simulink model "SrmAmLinearApcZhw3a1tst UNKnwn"  (R2013b)
settings: Solver=ode45  StartTime=0.0  StopTime=2  MaxStep=1e-4  RelTol=1e-3
InitFcn:
  | theta0=30*2*pi/360;
  | ks=2.44;
  | is=2;
  | lu=0.016;
  | rs=5;
  | lux=1;
  | j=1;
settings Model: Creator=mamingkai  LastModifiedBy=Think79

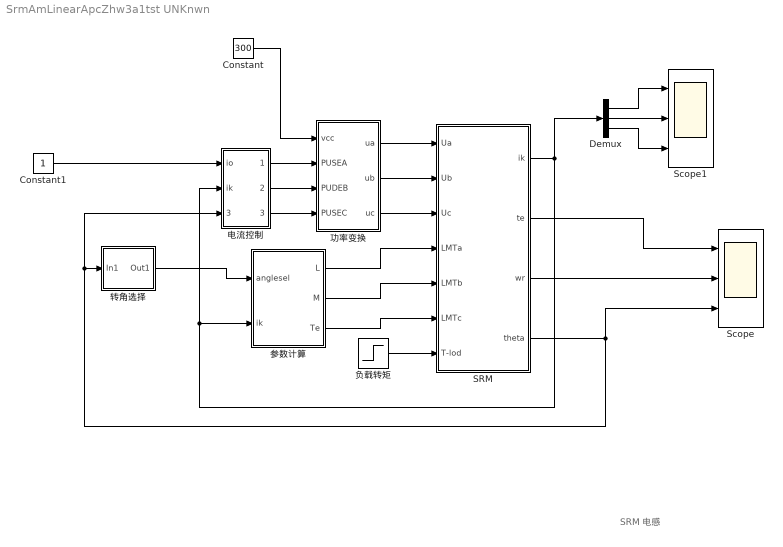
== system SrmAmLinearApcZhw3a1tst UNKnwn ==
  note: SRM 电感
  Constant : Constant  Value=300
  Constant1 : Constant
  Demux : Demux  Outputs=3
  SRM : Subsystem
  Scope : Scope  NumInputPorts=3
      settings: YMin=-5~-5~-5  YMax=5~5~5
  Scope1 : Scope  NumInputPorts=3
      settings: YMin=-5~-5~-5  YMax=5~5~5  SaveName=ScopeData6
  功率变换 : Subsystem
  参数计算 : Subsystem
  电流控制 : Subsystem
  负载转矩 : Step  After=0  SampleTime=0
  转角选择 : Subsystem
  wires:
  电流控制/1(Out1) -> 功率变换/2(PUSEA)
  电流控制/2(Out2) -> 功率变换/3(PUDEB)
  电流控制/3(Out3) -> 功率变换/4(PUSEC)
  Constant1/1 -> 电流控制/1(io)
  Constant/1 -> 功率变换/1(vcc)
  功率变换/1(ua) -> SRM/1(Ua)
  功率变换/2(ub) -> SRM/2(Ub)
  功率变换/3(uc) -> SRM/3(Uc)
  转角选择/1(Out1) -> 参数计算/1("anglesel ")
  SRM/1(ik) -> 电流控制/2(ik), 参数计算/2(ik), Demux/1
  SRM/3(wr) -> Scope/2
  SRM/4(theta) -> Scope/3, 电流控制/3(teta), 转角选择/1(In1)
  SRM/2(te) -> Scope/1
  参数计算/1(L) -> SRM/4(LMTa)
  参数计算/2(M) -> SRM/5(LMTb)
  参数计算/3(Te) -> SRM/6(LMTc)
  负载转矩/1 -> SRM/7(T-lod)
  Demux/1 -> Scope1/1
  Demux/2 -> Scope1/2
  Demux/3 -> Scope1/3

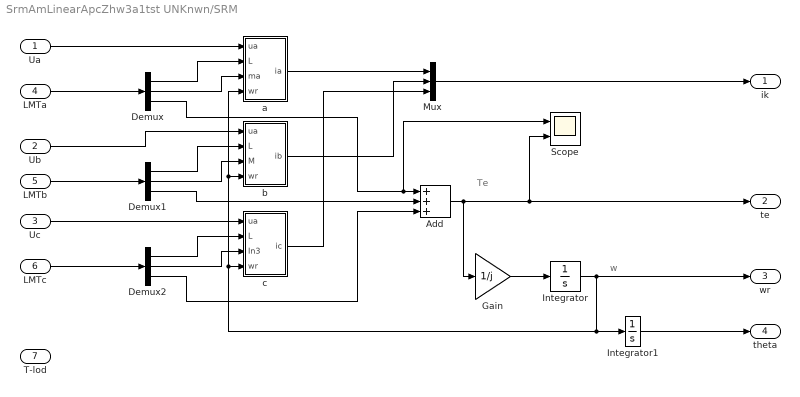
== system SrmAmLinearApcZhw3a1tst UNKnwn/SRM ==
  note: w
  note: Te
  Ua : Inport
  Ub : Inport  Port=2
  Uc : Inport  Port=3
  LMTa : Inport  Port=4
  LMTb : Inport  Port=5
  LMTc : Inport  Port=6
  T-lod : Inport  Port=7
  Add : Sum  Inputs=+++
  Demux : Demux  Outputs=3
  Demux1 : Demux  Outputs=3
  Demux2 : Demux  Outputs=3
  Gain : Gain  Gain=1/j
  Integrator : Integrator
  Integrator1 : Integrator
  Mux : Mux  Inputs=3
  Scope : Scope  NumInputPorts=2
      settings: YMin=-5~-5  YMax=5~5
  a : Subsystem
  b : Subsystem
  c : Subsystem
  ik : Outport
  te : Outport  Port=2
  wr : Outport  Port=3
  theta : Outport  Port=4
  wires:
  LMTa/1 -> Demux/1
  Demux/1 -> a/2("L ")
  Demux/2 -> a/3(ma)
  Demux/3 -> Scope/1, Add/1
  Ub/1 -> b/1(ua)
  Demux1/1 -> b/2(L)
  Demux1/2 -> b/3(M)
  Demux1/3 -> Add/2
  Uc/1 -> c/1(ua)
  LMTc/1 -> Demux2/1
  LMTb/1 -> Demux1/1
  Demux2/1 -> c/2(L)
  Demux2/2 -> c/3(In3)
  Demux2/3 -> Add/3
  Integrator/1 -> wr/1, c/4(wr), b/4("wr "), a/4(wr), Integrator1/1
  a/1(ia) -> Mux/1
  b/1("ib ") -> Mux/2
  c/1(ic) -> Mux/3
  Mux/1 -> ik/1
  Add/1 -> Gain/1, te/1, Scope/2
  Gain/1 -> Integrator/1
  Integrator1/1 -> theta/1
  Ua/1 -> a/1(ua)

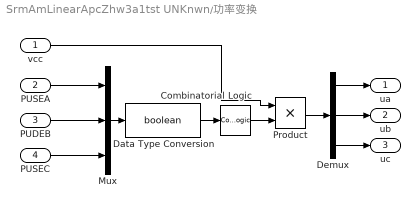
== system SrmAmLinearApcZhw3a1tst UNKnwn/功率变换 ==
  vcc : Inport
  PUSEA : Inport  Port=2
  PUDEB : Inport  Port=3
  PUSEC : Inport  Port=4
  Combinatorial Logic : CombinatorialLogic  TruthTable=[0 0 0 ;0 0 1;0 1 0;0 1 1;1 0 0;1 0 1;1 1 0;1 1 1]
  Data Type Conversion : DataTypeConversion  OutDataTypeStr=boolean
  Demux : Demux  Outputs=3
  Mux : Mux  Inputs=3
  Product : Product
  ua : Outport
  ub : Outport  Port=2
  uc : Outport  Port=3
  wires:
  PUSEA/1 -> Mux/1
  Demux/1 -> ua/1
  Product/1 -> Demux/1
  Demux/2 -> ub/1
  Demux/3 -> uc/1
  PUDEB/1 -> Mux/2
  PUSEC/1 -> Mux/3
  Combinatorial Logic/1 -> Product/2
  vcc/1 -> Product/1
  Mux/1 -> Data Type Conversion/1
  Data Type Conversion/1 -> Combinatorial Logic/1

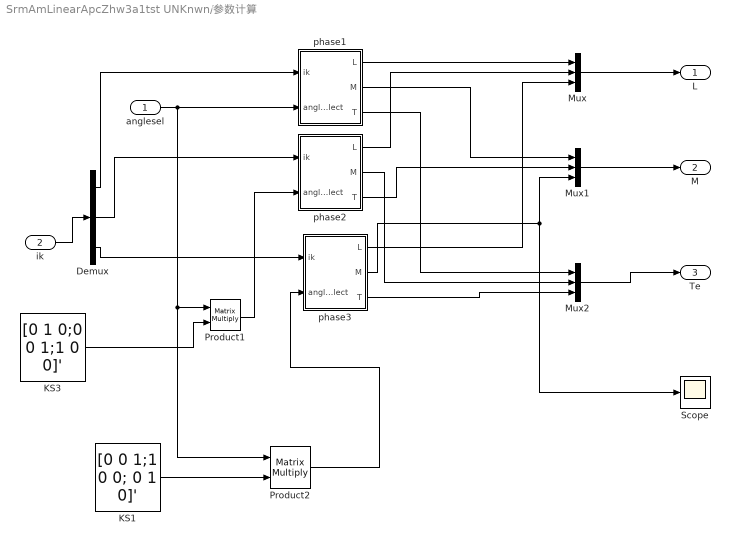
== system SrmAmLinearApcZhw3a1tst UNKnwn/参数计算 ==
  "anglesel " : Inport
  ik : Inport  Port=2
  Demux : Demux  Outputs=3
  KS1 : Constant  Value="[0 0 1;1 0  0; 0 1 0]'"  VectorParams1D=off
  KS3 : Constant  Value="[0 1 0;0  0 1;1 0 0]'"  VectorParams1D=off
  Mux : Mux  Inputs=3
  Mux1 : Mux  Inputs=3
  Mux2 : Mux  Inputs=3
  Product1 : Product  Multiplication=Matrix(*)
  Product2 : Product  Multiplication=Matrix(*)
  Scope : Scope
      settings: SaveName=ScopeData15
  phase1 : Subsystem
  phase2 : Subsystem
  phase3 : Subsystem
  L : Outport
  M : Outport  Port=2
  Te : Outport  Port=3
  wires:
  Mux/1 -> L/1
  "anglesel "/1 -> Product2/1, Product1/1, phase1/2("angleselect ")
  ik/1 -> Demux/1
  Demux/1 -> phase1/1(ik)
  Demux/2 -> phase2/1(ik)
  Demux/3 -> phase3/1(ik)
  phase1/1("L ") -> Mux/1
  phase1/2(M) -> Mux1/1
  phase1/3(T) -> Mux2/1
  phase2/1("L ") -> Mux/2
  phase2/3(T) -> Mux1/2
  phase2/2(M) -> Mux2/2
  phase3/1("L ") -> Mux/3
  phase3/2(M) -> Mux1/3, Scope/1
  phase3/3(T) -> Mux2/3
  Mux1/1 -> M/1
  Mux2/1 -> Te/1
  KS3/1 -> Product1/2
  Product1/1 -> phase2/2("angleselect ")
  KS1/1 -> Product2/2
  Product2/1 -> phase3/2("angleselect ")

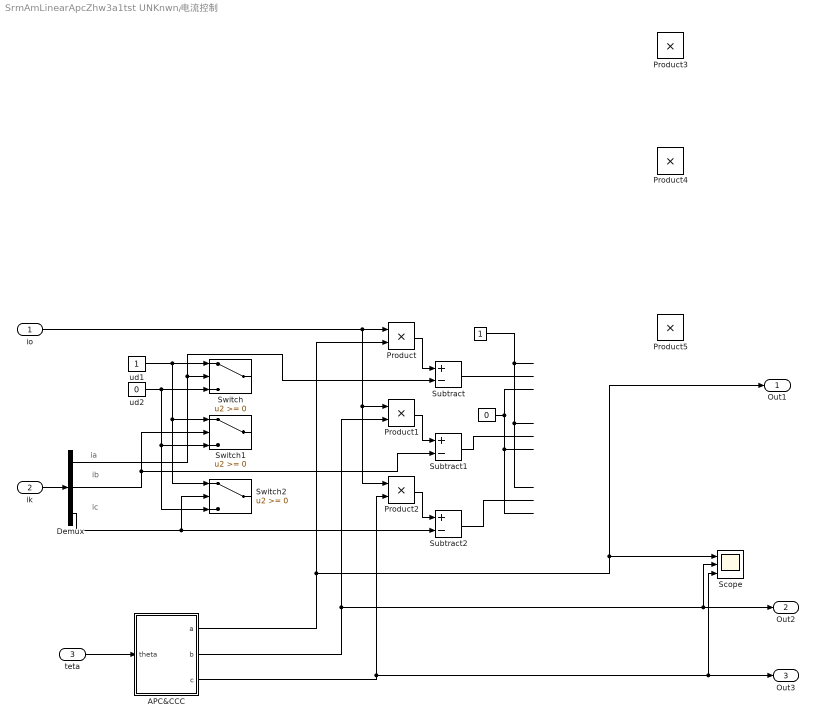
== system SrmAmLinearApcZhw3a1tst UNKnwn/电流控制 ==
  note: ic
  note: ib
  note: ia
  io : Inport
  ik : Inport  Port=2
  teta : Inport  Port=3
  " " : Constant
  " " : Constant  Value=0
  APC&CCC : Subsystem
  Demux : Demux  Outputs=3
  Product{,1..5} (6 alike) : Product
  Scope : Scope  NumInputPorts=3
      settings: YMin=-5~-5~-5  YMax=5~5~5  SaveName=ScopeData4
  Subtract : Sum  Inputs=+-
  Subtract1 : Sum  Inputs=+-
  Subtract2 : Sum  Inputs=+-
  Switch : Switch
  Switch1 : Switch
  Switch2 : Switch
  ud1 : Constant
  ud2 : Constant  Value=0
  Out1 : Outport
  Out2 : Outport  Port=2
  Out3 : Outport  Port=3
  wires:
  ik/1 -> Demux/1
  io/1 -> Product2/1, Product1/1, Product/1
  ud1/1 -> Switch2/1, Switch1/1, Switch/1
  ud2/1 -> Switch2/3, Switch1/3, Switch/3
  teta/1 -> APC&CCC/1(theta)
  Demux/1 -> Subtract/2, Switch/2
  Demux/3 -> Switch2/2, Subtract2/2
  Demux/2 -> Switch1/2, Subtract1/2
  APC&CCC/1(a) -> Out1/1, Scope/1, Product/2
  Product/1 -> Subtract/1
  Product1/1 -> Subtract1/1
  Product2/1 -> Subtract2/1
  " "/1 -> ?
  " "/1 -> ?
  ? -> Product5/1
  ? -> Product4/1
  ? -> Product3/1
  APC&CCC/3(c) -> Scope/3, Out3/1, Product2/2
  Subtract1/1 -> ?
  Subtract/1 -> ?
  Subtract2/1 -> ?
  APC&CCC/2(b) -> Scope/2, Out2/1, Product1/2

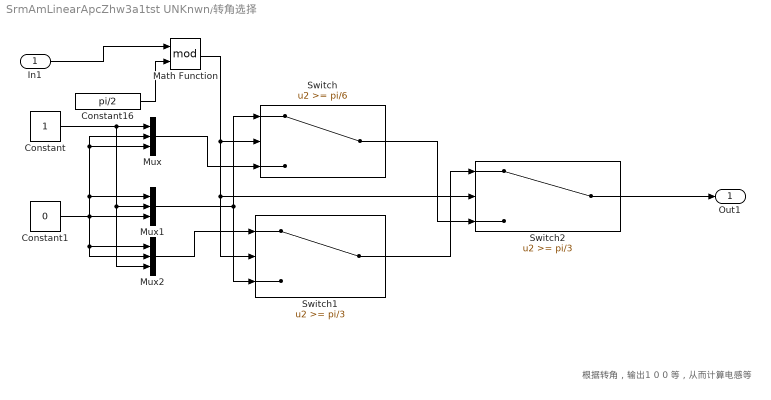
== system SrmAmLinearApcZhw3a1tst UNKnwn/转角选择 ==
  note: 根据转角，输出1 0 0 等，从而计算电感等
  In1 : Inport
  Constant : Constant
  Constant1 : Constant  Value=0
  Constant16 : Constant  Value=pi/2
  Math Function : Math  Operator=mod  SaturateOnIntegerOverflow=on
  Mux : Mux  Inputs=3
  Mux1 : Mux  Inputs=3
  Mux2 : Mux  Inputs=3
  Switch : Switch  Threshold=pi/6
  Switch1 : Switch  Threshold=pi/3
  Switch2 : Switch  Threshold=pi/3
  Out1 : Outport
  wires:
  In1/1 -> Math Function/1
  Constant/1 -> Mux2/3, Mux1/2, Mux/1
  Mux/1 -> Switch/3
  Constant1/1 -> Mux/3, Mux/2, Mux1/1, Mux2/2, Mux2/1, Mux1/3
  Mux1/1 -> Switch1/3, Switch/1
  Mux2/1 -> Switch1/1
  Math Function/1 -> Switch2/2, Switch1/2, Switch/2
  Switch/1 -> Switch2/3
  Switch1/1 -> Switch2/1
  Switch2/1 -> Out1/1
  Constant16/1 -> Math Function/2

== system SrmAmLinearApcZhw3a1tst UNKnwn/SRM/a ==
  ua : Inport
  "L " : Inport  Port=2
  ma : Inport  Port=3
  wr : Inport  Port=4
  Add : Sum  Inputs=+--
  Constant : Constant  Value=lux
  Gain : Gain  Gain=rs
  Integrator : Integrator
  Product : Product
  Product1 : Product
  Scope : Scope
      settings: SaveName=ScopeData2
  ia : Outport
  wires:
  wr/1 -> Product/2
  Integrator/1 -> Scope/1, Gain/1, ia/1
  ma/1 -> Product/1
  ua/1 -> Add/1
  Gain/1 -> Add/2
  Product/1 -> Add/3
  Add/1 -> Product1/1
  Product1/1 -> Integrator/1
  "L "/1 -> ?
  Constant/1 -> Product1/2

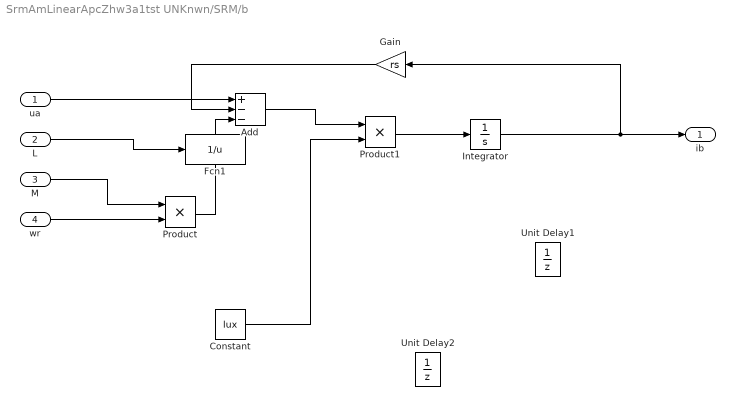
== system SrmAmLinearApcZhw3a1tst UNKnwn/SRM/b ==
  ua : Inport
  L : Inport  Port=2
  M : Inport  Port=3
  "wr " : Inport  Port=4
  Add : Sum  Inputs=+--
  Constant : Constant  Value=lux
  Fcn1 : Fcn  Expr=1/u
  Gain : Gain  Gain=rs
  Integrator : Integrator
  Product : Product
  Product1 : Product
  Unit Delay1 : UnitDelay  SampleTime=-1
  Unit Delay2 : UnitDelay  SampleTime=-1
  "ib " : Outport
  wires:
  "wr "/1 -> Product/2
  M/1 -> Product/1
  ua/1 -> Add/1
  Gain/1 -> Add/2
  Product/1 -> Add/3
  Add/1 -> Product1/1
  Product1/1 -> Integrator/1
  Integrator/1 -> Gain/1, "ib "/1
  L/1 -> Fcn1/1
  Constant/1 -> Product1/2

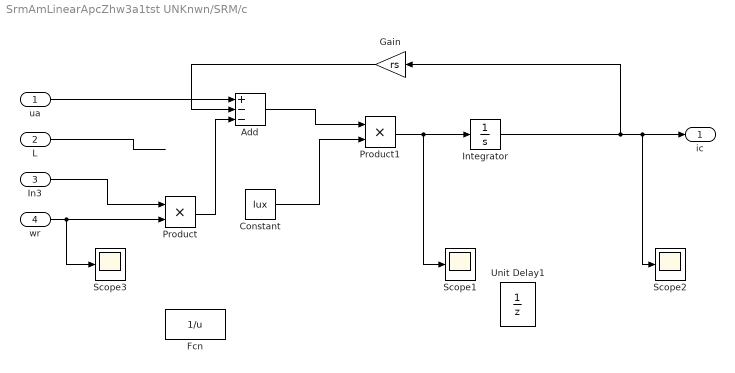
== system SrmAmLinearApcZhw3a1tst UNKnwn/SRM/c ==
  ua : Inport
  L : Inport  Port=2
  In3 : Inport  Port=3
  wr : Inport  Port=4
  Add : Sum  Inputs=+--
  Constant : Constant  Value=lux
  Fcn : Fcn  Expr=1/u
  Gain : Gain  Gain=rs
  Integrator : Integrator  InitialCondition=1e-5
  Product : Product
  Product1 : Product
  Scope1 : Scope
      settings: TimeRange=2  YMin=-1  YMax=1  SaveName=ScopeData13
  Scope2 : Scope
      settings: TimeRange=2  YMin=-1  YMax=1  SaveName=ScopeData12
  Scope3 : Scope
      settings: TimeRange=2  YMin=-1  YMax=1  SaveName=ScopeData14
  Unit Delay1 : UnitDelay  SampleTime=-1
  ic : Outport
  wires:
  wr/1 -> Scope3/1, Product/2
  In3/1 -> Product/1
  ua/1 -> Add/1
  Gain/1 -> Add/2
  Product/1 -> Add/3
  Add/1 -> Product1/1
  Integrator/1 -> Gain/1, Scope2/1, ic/1
  Product1/1 -> Scope1/1, Integrator/1
  L/1 -> ?
  Constant/1 -> Product1/2

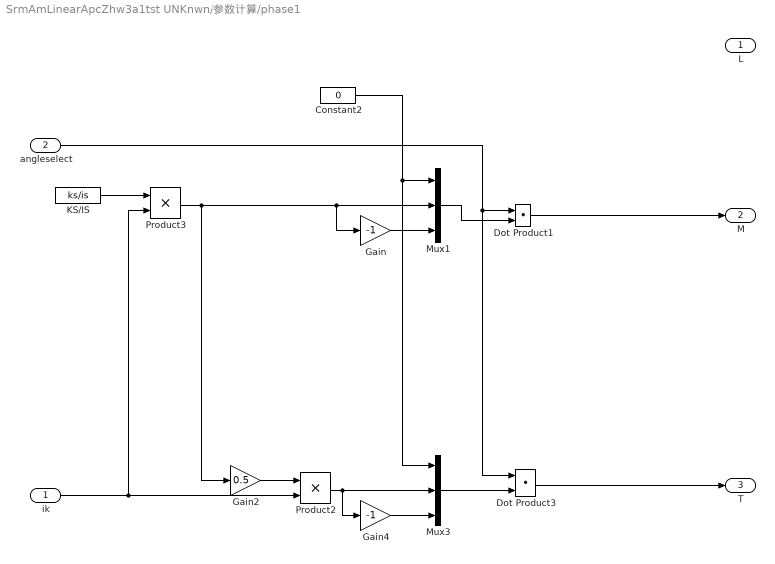
== system SrmAmLinearApcZhw3a1tst UNKnwn/参数计算/phase1 ==
  ik : Inport
  "angleselect " : Inport  Port=2
  Constant2 : Constant  Value=0
  Dot Product1 : DotProduct  InputSameDT=on  OutDataTypeStr=Inherit: Inherit via internal rule
  Dot Product3 : DotProduct  InputSameDT=on  OutDataTypeStr=Inherit: Inherit via internal rule
  Gain : Gain  Gain=-1
  Gain2 : Gain  Gain=0.5
  Gain4 : Gain  Gain=-1
  KS/IS : Constant  Value=ks/is
  Mux1 : Mux  Inputs=3
  Mux3 : Mux  Inputs=3
  Product2 : Product
  Product3 : Product
  "L " : Outport
  M : Outport  Port=2
  T : Outport  Port=3
  wires:
  ? -> "L "/1
  KS/IS/1 -> Product3/1
  ik/1 -> Product3/2, Product2/2
  "angleselect "/1 -> Dot Product3/1, Dot Product1/1
  Constant2/1 -> Mux3/1, Mux1/1
  Mux3/1 -> Dot Product3/2
  Mux1/1 -> Dot Product1/2
  Product3/1 -> Gain/1, Mux1/2, Gain2/1
  Gain/1 -> Mux1/3
  Gain2/1 -> Product2/1
  Dot Product1/1 -> M/1
  Dot Product3/1 -> T/1
  Product2/1 -> Gain4/1, Mux3/2
  Gain4/1 -> Mux3/3

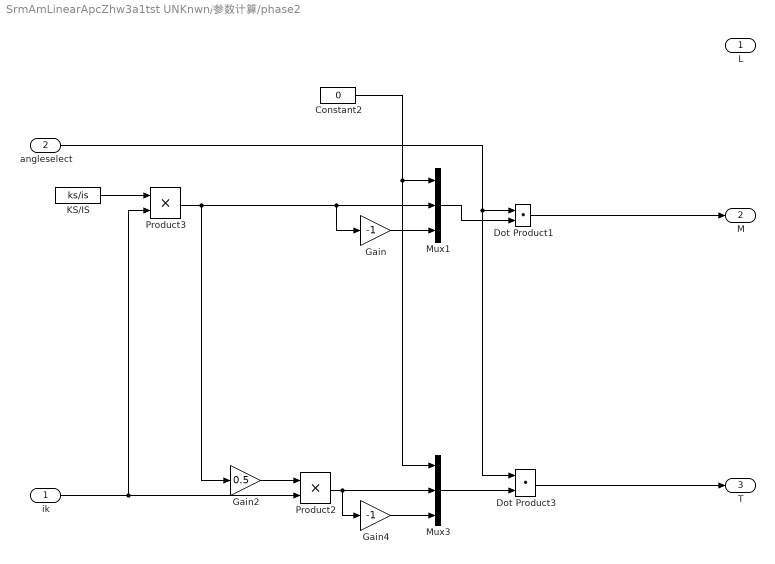
== system SrmAmLinearApcZhw3a1tst UNKnwn/参数计算/phase2 ==
  ik : Inport
  "angleselect " : Inport  Port=2
  Constant2 : Constant  Value=0
  Dot Product1 : DotProduct  InputSameDT=on  OutDataTypeStr=Inherit: Inherit via internal rule
  Dot Product3 : DotProduct  InputSameDT=on  OutDataTypeStr=Inherit: Inherit via internal rule
  Gain : Gain  Gain=-1
  Gain2 : Gain  Gain=0.5
  Gain4 : Gain  Gain=-1
  KS/IS : Constant  Value=ks/is
  Mux1 : Mux  Inputs=3
  Mux3 : Mux  Inputs=3
  Product2 : Product
  Product3 : Product
  "L " : Outport
  M : Outport  Port=2
  T : Outport  Port=3
  wires:
  Gain4/1 -> Mux3/3
  Product2/1 -> Mux3/2, Gain4/1
  Dot Product3/1 -> T/1
  Dot Product1/1 -> M/1
  Gain2/1 -> Product2/1
  Gain/1 -> Mux1/3
  Product3/1 -> Gain2/1, Mux1/2, Gain/1
  Mux1/1 -> Dot Product1/2
  Mux3/1 -> Dot Product3/2
  Constant2/1 -> Mux1/1, Mux3/1
  "angleselect "/1 -> Dot Product1/1, Dot Product3/1
  ik/1 -> Product2/2, Product3/2
  KS/IS/1 -> Product3/1
  ? -> "L "/1

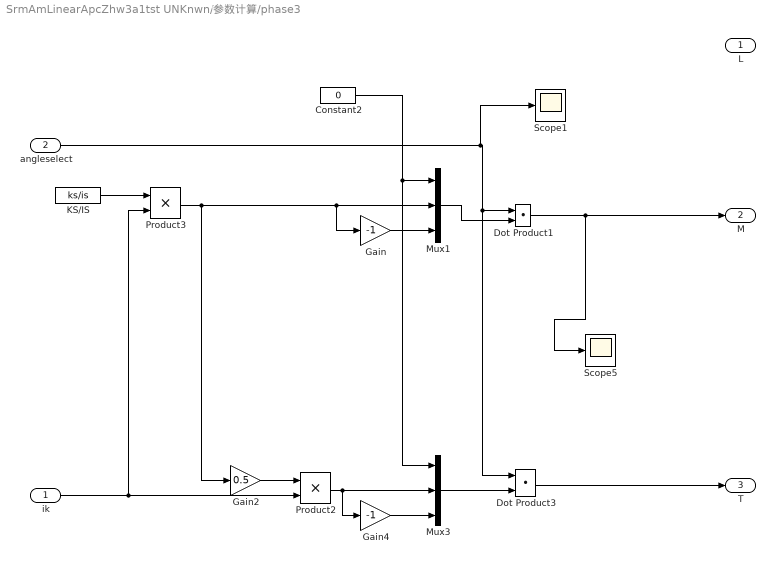
== system SrmAmLinearApcZhw3a1tst UNKnwn/参数计算/phase3 ==
  ik : Inport
  "angleselect " : Inport  Port=2
  Constant2 : Constant  Value=0
  Dot Product1 : DotProduct  InputSameDT=on  OutDataTypeStr=Inherit: Inherit via internal rule
  Dot Product3 : DotProduct  InputSameDT=on  OutDataTypeStr=Inherit: Inherit via internal rule
  Gain : Gain  Gain=-1
  Gain2 : Gain  Gain=0.5
  Gain4 : Gain  Gain=-1
  KS/IS : Constant  Value=ks/is
  Mux1 : Mux  Inputs=3
  Mux3 : Mux  Inputs=3
  Product2 : Product
  Product3 : Product
  Scope1 : Scope
      settings: TimeRange=2  YMin=-1  YMax=1  SaveName=ScopeData17
  Scope5 : Scope
      settings: TimeRange=2  YMin=-1  YMax=1  SaveName=ScopeData16
  "L " : Outport
  M : Outport  Port=2
  T : Outport  Port=3
  wires:
  ? -> "L "/1
  KS/IS/1 -> Product3/1
  ik/1 -> Product3/2, Product2/2
  "angleselect "/1 -> Scope1/1, Dot Product3/1, Dot Product1/1
  Constant2/1 -> Mux3/1, Mux1/1
  Mux3/1 -> Dot Product3/2
  Mux1/1 -> Dot Product1/2
  Product3/1 -> Gain/1, Mux1/2, Gain2/1
  Gain/1 -> Mux1/3
  Gain2/1 -> Product2/1
  Dot Product1/1 -> Scope5/1, M/1
  Dot Product3/1 -> T/1
  Product2/1 -> Gain4/1, Mux3/2
  Gain4/1 -> Mux3/3

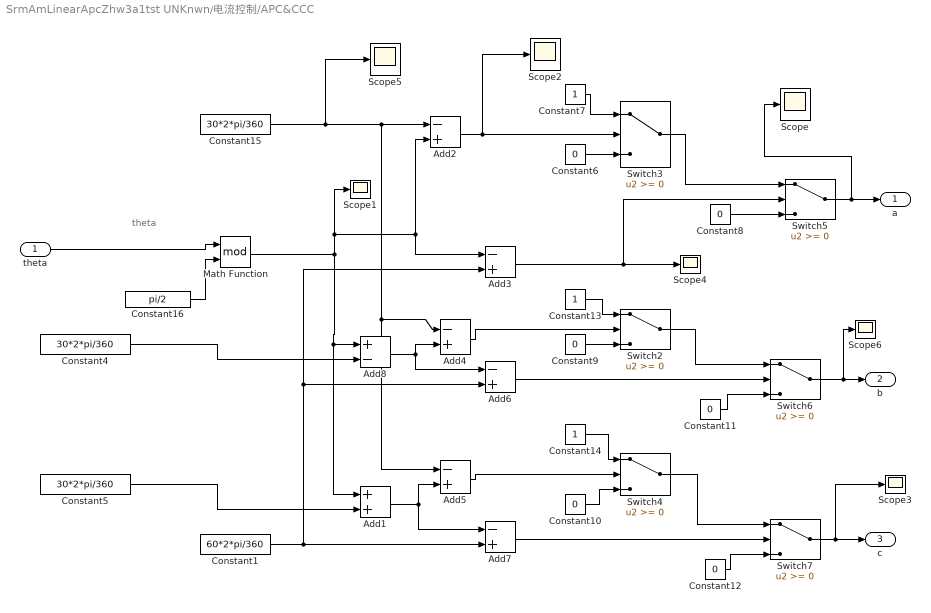
== system SrmAmLinearApcZhw3a1tst UNKnwn/电流控制/APC&CCC ==
  note: theta
  theta : Inport
  Add1 : Sum
  Add{2..7} (6 alike) : Sum  Inputs=-+
  Add8 : Sum  Inputs=+-
  Constant1 : Constant  Value=60*2*pi/360
  Constant{6,8..12} (6 alike) : Constant  Value=0
  Constant13 : Constant
  Constant14 : Constant
  Constant15 : Constant  Value=30*2*pi/360
  Constant16 : Constant  Value=pi/2
  Constant4 : Constant  Value=30*2*pi/360
  Constant5 : Constant  Value=30*2*pi/360
  Constant7 : Constant
  Math Function : Math  Operator=mod  SaturateOnIntegerOverflow=on
  Scope{,1..6} (7 alike) : Scope
      Scope settings: TimeRange=2  YMin=-1  YMax=1  SaveName=ScopeData3
      Scope1 settings: SaveName=ScopeData5
      Scope2 settings: TimeRange=2  YMin=-1  YMax=1  SaveName=ScopeData7
      Scope3 settings: SaveName=ScopeData8
      Scope4 settings: SaveName=ScopeData9
      Scope5 settings: TimeRange=2  YMin=-1  YMax=1  SaveName=ScopeData10
      Scope6 settings: SaveName=ScopeData11
  Switch{2..7} (6 alike) : Switch
  a : Outport
  b : Outport  Port=2
  c : Outport  Port=3
  wires:
  Switch5/1 -> Scope/1, a/1
  Constant1/1 -> Add3/2, Add6/2, Add7/2
  Constant15/1 -> Scope5/1, Add5/1, Add4/1, Add2/1
  theta/1 -> Math Function/1
  Add3/1 -> Switch5/2, Scope4/1
  Add6/1 -> Switch6/2
  Add7/1 -> Switch7/2
  Constant6/1 -> Switch3/3
  Switch3/1 -> Switch5/1
  Switch2/1 -> Switch6/1
  Switch4/1 -> Switch7/1
  Switch6/1 -> Scope6/1, b/1
  Switch7/1 -> Scope3/1, c/1
  Add2/1 -> Scope2/1, Switch3/2
  Constant12/1 -> Switch7/3
  Constant11/1 -> Switch6/3
  Constant10/1 -> Switch4/3
  Constant9/1 -> Switch2/3
  Constant8/1 -> Switch5/3
  Constant7/1 -> Switch3/1
  Constant13/1 -> Switch2/1
  Constant14/1 -> Switch4/1
  Add5/1 -> Switch4/2
  Add4/1 -> Switch2/2
  Math Function/1 -> Scope1/1, Add3/1, Add2/2, Add8/1, Add1/1
  Constant16/1 -> Math Function/2
  Constant5/1 -> Add1/2
  Add1/1 -> Add5/2, Add7/1
  Constant4/1 -> Add8/2
  Add8/1 -> Add6/1, Add4/2
